simulink model "Lab1_2_simple"  (Simulink 8.0)
settings: Solver=ode3  StartTime=0.0  StopTime=10.0  FixedStep=0.001  RelTol=1e-3
undefined symbols (not defined in the file or in its folder): MultiQ, PCI, Quanser
libraries: rtwinlib x3
settings Model: Creator=Mehatronicki Sustavi  LastModifiedBy=Niko  SimulationMode=external  ExtModeTrigDuration=1000000
settings DataIOCC: SignalLoggingSaveFormat=ModelDataLogs
settings DebuggingCC: FcnCallInpInsideContextMsg=UseLocalSettings  StrictBusMsg=Warning
settings HardwareCC: ProdIntDivRoundTo=Zero  ProdEndianess=LittleEndian  ProdHWDeviceType=Generic->32-bit x86 compatible
settings RTWCC: SystemTargetFile=rtwin.tlc  TemplateMakefile=rtwin.tmf  Description=Real-Time Windows Target  ProcessScript=rtwin_make_rtw_hook  RTWCompilerOptimization=On
settings CodeAppCC: MaxIdLength=95
settings RTWinTargetCC: TargetLibSuffix=_rtwin.lib  TargetPreCompLibLocation=G:\Program Files\MATLAB\R2012b\toolbox\rtw\targets\rtwin\lib\win64  CodeReplacementLibrary=ANSI_C  RTWinDir=G:/Program Files/MATLAB/R2012b/toolbox/rtw/targets/rtwin  TargetArch=win64

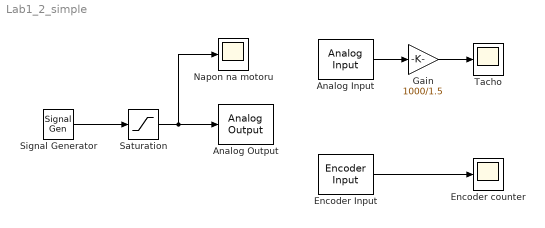
== system Lab1_2_simple ==
  Analog Input : rtwinlib/Analog Input  SampleTime=0.001  MaxMissedTicks=10  ShowMissedTicks=off  YieldWhenWaiting=off  DrvName=Quanser/MultiQ-PCI  DrvAddress=4294967295  DrvOptions=zeros(1,0)  Channels=2  RangeMode=1  VoltRange=1  DataType=1
      settings: AttributesFormatString=Quanser\nMultiQ-PCI [auto]
  Analog Output : rtwinlib/Analog Output  SampleTime=0.001  MaxMissedTicks=10  ShowMissedTicks=off  YieldWhenWaiting=off  DrvName=Quanser/MultiQ-PCI  DrvAddress=4294967295  DrvOptions=zeros(1,0)  Channels=1  RangeMode=1  VoltRange=1  InitialValue=0  FinalValue=0
      settings: AttributesFormatString=Quanser\nMultiQ-PCI [auto]
  Encoder Input : rtwinlib/Encoder Input  SampleTime=0.001  MaxMissedTicks=10  ShowMissedTicks=off  YieldWhenWaiting=off  DrvName=Quanser/MultiQ-PCI  DrvAddress=4294967295  DrvOptions=zeros(1,0)  Channels=1  QuadMode=3  IndexPulse=2  InputFilter=Inf  DataType=1
      settings: AttributesFormatString=Quanser\nMultiQ-PCI [auto]
  Encoder counter : Scope
      settings: YMin=0  YMax=12000  SaveName=EncoderCnt
  Gain : Gain  Gain=1000/1.5
  Napon na motoru : Scope
      settings: SaveName=NaponMotor
  Saturation : Saturate  UpperLimit=6  LowerLimit=-6
  Signal Generator : SignalGenerator  WaveForm=square  Amplitude=3  Frequency=0.1
  Tacho : Scope
      settings: YMin=-3500  YMax=3500  SaveName=Tacho
  wires:
  Signal Generator/1 -> Saturation/1
  Saturation/1 -> Analog Output/1, Napon na motoru/1
  Analog Input/1 -> Gain/1
  Gain/1 -> Tacho/1
  Encoder Input/1 -> Encoder counter/1
